simulink model "IEEE13NodeTestFeeder"  (R2023b)
settings: Solver=FixedStepAuto  StartTime=0.0  StopTime=3  FixedStep=0.004  MaxStep=0.04  RelTol=1e-3
PreLoadFcn:
  | IEEE13NodeTestFeederInit;
  | Ts=50e-6;
values from neighbouring files (symbols this model uses):
  C_601 = B_601/mi2km*ms2F    [IEEE13NodeTestFeederInit.m]
  C_602 = B_602/mi2km*ms2F    [IEEE13NodeTestFeederInit.m]
  C_603 = B_603/mi2km*ms2F    [IEEE13NodeTestFeederInit.m]
  C_604 = B_604/mi2km*ms2F    [IEEE13NodeTestFeederInit.m]
  C_605 = B_605/mi2km*ms2F    [IEEE13NodeTestFeederInit.m]
  C_606 = B_606/mi2km*ms2F    [IEEE13NodeTestFeederInit.m]
  C_607 = B_607/mi2km*ms2F    [IEEE13NodeTestFeederInit.m]
  ft2km = 0.0003048    [IEEE13NodeTestFeederInit.m]
  L_601 = X_601/mi2km/2/pi/60    [IEEE13NodeTestFeederInit.m]
  L_602 = X_602/mi2km/2/pi/60    [IEEE13NodeTestFeederInit.m]
  L_603 = X_603/mi2km/2/pi/60    [IEEE13NodeTestFeederInit.m]
  L_604 = X_604/mi2km/2/pi/60    [IEEE13NodeTestFeederInit.m]
  L_605 = X_605/mi2km/2/pi/60    [IEEE13NodeTestFeederInit.m]
  L_606 = X_606/mi2km/2/pi/60    [IEEE13NodeTestFeederInit.m]
  L_607 = X_607/mi2km/2/pi/60    [IEEE13NodeTestFeederInit.m]
  R_601 = R_601/mi2km    [IEEE13NodeTestFeederInit.m]
  R_602 = R_602/mi2km    [IEEE13NodeTestFeederInit.m]
  R_603 = R_603/mi2km    [IEEE13NodeTestFeederInit.m]
  R_604 = R_604/mi2km    [IEEE13NodeTestFeederInit.m]
  R_605 = R_605/mi2km    [IEEE13NodeTestFeederInit.m]
  R_606 = R_606/mi2km    [IEEE13NodeTestFeederInit.m]
  R_607 = R_607/mi2km    [IEEE13NodeTestFeederInit.m]
libraries: spsPowerPhasorLib x18, spsThreePhaseVIMeasurementLib x16, spsSeriesRLCLoadLib x12, spsLoadFlowBusLib x12, spsThreePhaseFaultLib x12, spsGroundLib x10, spsPiSectionLineLib x9, spsThreePhaseSeriesRLCLoadLib x8, spsMultimeterLib x6, spsThreePhaseSourceLib x1, spsThreePhaseBreakerLib x1, spsThreePhaseTransformerTwoWindingsLib x1
settings Model: Creator=The MathWorks, Inc.  LastModifiedBy=Dell
settings SolverCC: AlgebraicLoopSolver=TrustRegion
settings DataIOCC: ExternalInput=getinputstruct(op_IEEE_13_node_5)  InitialState=getstatestruct(op_IEEE_13_node_5)  LimitDataPoints=on  SaveFinalState=on  SaveOperatingPoint=on  SaveFormat=StructureWithTime  SaveState=on  LoggingToFile=on
settings OptimizationCC: LifeSpan=inf
settings DebuggingCC: AlgebraicLoopMsg=none  FcnCallInpInsideContextMsg=warning  StateNameClashWarn=warning  SFUnexpectedBacktrackingDiag=warning  SFNoUnconditionalDefaultTransitionDiag=warning  SFExecutionAtInitializationDiag=none
settings ModelReferenceCC: EnableRefExpFcnMdlSchedulingChecks=on  PropagateSignalLabelsOutOfModel=off
settings SFSimCC: CustomCodeUndefinedFunction=UseInterfaceOnly
settings CodeAppCC: StateflowObjectComments=on
settings SimscapeCC: SimscapeNormalizeSystem=off

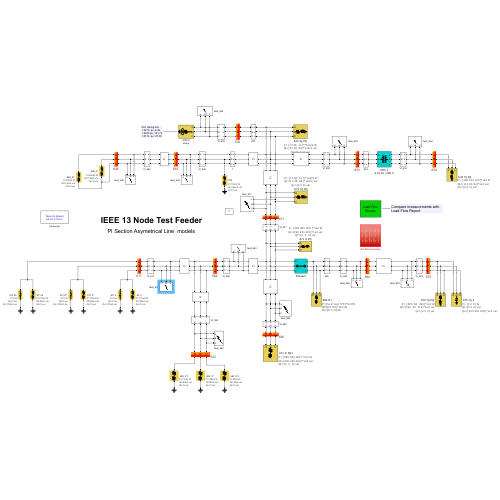
[thumbnail: Simulink's stored preview of the top-level diagram]
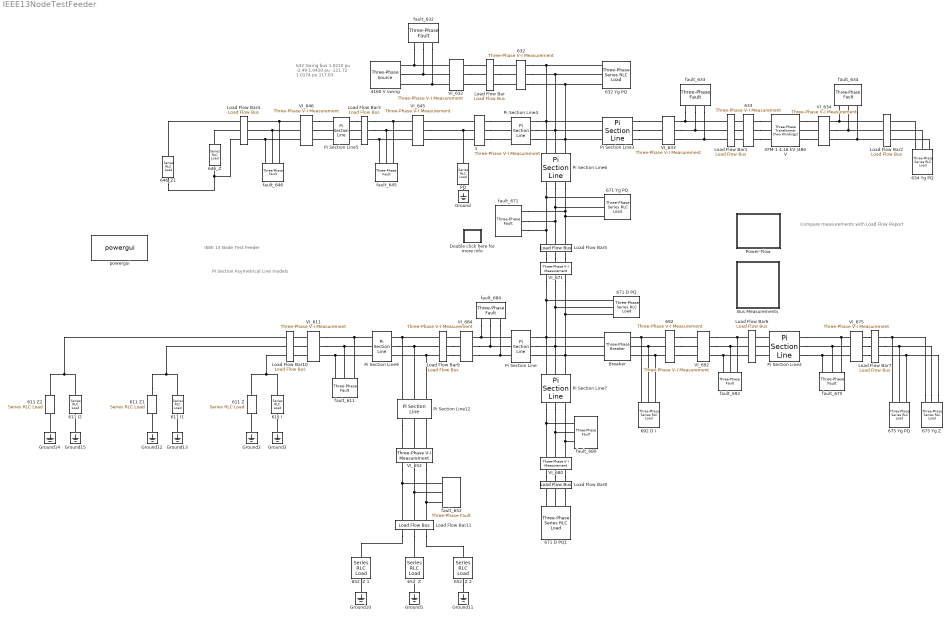
== system IEEE13NodeTestFeeder ==
  note: Compare measurements with
      | Load Flow Report
  note: 632 Swing bus
      | 1.0210 pu -2.49
      | 1.0420 pu -121.72
      | 1.0174 pu 117.83
  note: PI Section Asymetrical Line models
  note: IEEE 13 Node Test Feeder
  " 634 Yg PQ " : spsThreePhaseSeriesRLCLoadLib/Three-Phase Series RLC Load  LConnTagsString=A|B|C  Configuration=Y (grounded)  NominalVoltage=120e3  Vabc=[ 0.993926 1.02168 0.995885]*277.128  Vabcp=[1e3 1e3 1e3]  NominalFrequency=60  UnbalancedPower=on  ActivePower=1e+006  InductivePower=0  CapacitivePower=0  Pabc=[160 120 120]*1e3  QLabc=[110 90 90]*1e3  QCabc=[0 0 0]  Pabcp=[10e3 9e3 11e3]  QLabcp=[100 90 110]  QCabcp=[100 90 110]  Measurements=None  LoadType=constant PQ
      settings: AttributesFormatString=|
      | P= %<Pabc> W
      | Ql=%<QLabc> var
      | Qc=%<QCabc> var
  1 : spsThreePhaseVIMeasurementLib/Three-Phase V-I Measurement  VoltageMeasurement=phase-to-ground  SetLabelV=on  LabelV=Vabc_645  Vpu=off  VpuLL=off  CurrentMeasurement=yes  SetLabelI=on  LabelI=Iabc_645  Ipu=off  Pbase=100e6  Vbase=4160  OutputType=Complex  PhasorSimulation=on  PSBequivalent=0
  4160 V swing : spsThreePhaseSourceLib/Three-Phase Source  InternalConnection=Yg  VoltagePhases=on  Voltage=120e3  PhaseAngle=0  Voltage_phases=[ 1.021 1.042 1.0174]*2401.78  PhaseAngles_phases=[ -2.49006 -121.72 117.83]  Frequency=60  NonIdealSource=on  SpecifyImpedance=off  Resistance=1e-5  Inductance=0  ShortCircuitLevel=100e6  BaseVoltage=120e3  XRratio=10  BusType=swing  Pref=0  Qref=0  Prefabc=[0 0 0]  Qrefabc=[0 0 0]  Qmin="[-inf  -inf -inf]"  Qmax="[inf  inf inf]"
  611 I : spsSeriesRLCLoadLib/Series RLC Load  LConnTagsString=a  RConnTagsString=__new0  NominalVoltage=0.986755*2401.78  NominalFrequency=60  ActivePower=170e3  InductivePower=80e3  CapacitivePower=0  Setx0=off  InitialVoltage=0  SetiL0=off  InitialCurrent=0  Measurements=Branch voltage and current  LoadType=constant I
      settings: AttributesFormatString=|
      | P=%<ActivePower> W
      | Ql=%<InductivePower> var
      | Qc=%<CapacitivePower> var
  611 I1 : spsSeriesRLCLoadLib/Series RLC Load  LConnTagsString=a  RConnTagsString=__new0  NominalVoltage=0.986755*2401.78  NominalFrequency=60  ActivePower=170e3  InductivePower=80e3  CapacitivePower=0  Setx0=off  InitialVoltage=0  SetiL0=off  InitialCurrent=0  Measurements=Branch voltage and current  LoadType=constant PQ
      settings: AttributesFormatString=|
      | P=%<ActivePower> W
      | Ql=%<InductivePower> var
      | Qc=%<CapacitivePower> var
  611 I2 : spsSeriesRLCLoadLib/Series RLC Load  LConnTagsString=a  RConnTagsString=__new0  NominalVoltage=0.986755*2401.78  NominalFrequency=60  ActivePower=170e3  InductivePower=80e3  CapacitivePower=0  Setx0=off  InitialVoltage=0  SetiL0=off  InitialCurrent=0  Measurements=Branch voltage and current  LoadType=constant I
      settings: AttributesFormatString=|
      | P=%<ActivePower> W
      | Ql=%<InductivePower> var
      | Qc=%<CapacitivePower> var
  611 Z : spsSeriesRLCLoadLib/Series RLC Load  LConnTagsString=a  RConnTagsString=__new0  NominalVoltage=4160/sqrt(3)  NominalFrequency=60  ActivePower=0  InductivePower=0  CapacitivePower=100e3  Setx0=off  InitialVoltage=0  SetiL0=off  InitialCurrent=0  Measurements=None  LoadType=constant Z
      settings: AttributesFormatString=|
      | P=%<ActivePower> W
      | Ql=%<InductivePower> var
      | Qc=%<CapacitivePower> var
  611 Z1 : spsSeriesRLCLoadLib/Series RLC Load  LConnTagsString=a  RConnTagsString=__new0  NominalVoltage=4160/sqrt(3)  NominalFrequency=60  ActivePower=0  InductivePower=0  CapacitivePower=100e3  Setx0=off  InitialVoltage=0  SetiL0=off  InitialCurrent=0  Measurements=None  LoadType=constant I
      settings: AttributesFormatString=|
      | P=%<ActivePower> W
      | Ql=%<InductivePower> var
      | Qc=%<CapacitivePower> var
  611 Z2 : spsSeriesRLCLoadLib/Series RLC Load  LConnTagsString=a  RConnTagsString=__new0  NominalVoltage=4160/sqrt(3)  NominalFrequency=60  ActivePower=0  InductivePower=0  CapacitivePower=100e3  Setx0=off  InitialVoltage=0  SetiL0=off  InitialCurrent=0  Measurements=None  LoadType=constant PQ
      settings: AttributesFormatString=|
      | P=%<ActivePower> W
      | Ql=%<InductivePower> var
      | Qc=%<CapacitivePower> var
  632 : spsThreePhaseVIMeasurementLib/Three-Phase V-I Measurement  VoltageMeasurement=phase-to-ground  SetLabelV=on  LabelV=Vabc_632  Vpu=off  VpuLL=off  CurrentMeasurement=yes  SetLabelI=on  LabelI=Iabc_632  Ipu=off  Pbase=100e6  Vbase=4160  OutputType=Complex  PhasorSimulation=on  PSBequivalent=0
  632 Yg PQ : spsThreePhaseSeriesRLCLoadLib/Three-Phase Series RLC Load  LConnTagsString=A|B|C  Configuration=Y (grounded)  NominalVoltage=120e3  Vabc=[ 1.021 1.042 1.0174]*2401.78  Vabcp=[1e3 1e3 1e3]  NominalFrequency=60  UnbalancedPower=on  ActivePower=1e+006  InductivePower=0  CapacitivePower=0  Pabc="[17 66  117]*1e3/2"  QLabc="[10 38  68]*1e3/2"  QCabc=[0 0 0]  Pabcp=[10e3 9e3 11e3]  QLabcp=[100 90 110]  QCabcp=[100 90 110]  Measurements=None  LoadType=constant PQ
      settings: AttributesFormatString=|
      | P= %<Pabc> W
      | Ql=%<QLabc> var
      | Qc=%<QCabc> var
  633 : spsThreePhaseVIMeasurementLib/Three-Phase V-I Measurement  VoltageMeasurement=phase-to-ground  SetLabelV=on  LabelV=Vabc_633  Vpu=off  VpuLL=off  CurrentMeasurement=yes  SetLabelI=on  LabelI=Iabc_633  Ipu=off  Pbase=100e6  Vbase=4160  OutputType=Complex  PhasorSimulation=on  PSBequivalent=0
  646_Z : spsSeriesRLCLoadLib/Series RLC Load  LConnTagsString=a  RConnTagsString=__new0  NominalVoltage=4160  NominalFrequency=60  ActivePower=230e3  InductivePower=132e3  CapacitivePower=0  Setx0=off  InitialVoltage=0  SetiL0=off  InitialCurrent=0  Measurements=None  LoadType=constant Z
      settings: AttributesFormatString=|
      | P=%<ActivePower> W
      | Ql=%<InductivePower> var
      | Qc=%<CapacitivePower> var
  646_Z1 : spsSeriesRLCLoadLib/Series RLC Load  LConnTagsString=a  RConnTagsString=__new0  NominalVoltage=4160  NominalFrequency=60  ActivePower=230e3  InductivePower=132e3  CapacitivePower=0  Setx0=off  InitialVoltage=0  SetiL0=off  InitialCurrent=0  Measurements=None  LoadType=constant PQ
      settings: AttributesFormatString=|
      | P=%<ActivePower> W
      | Ql=%<InductivePower> var
      | Qc=%<CapacitivePower> var
  "652  Z " : spsSeriesRLCLoadLib/Series RLC Load  LConnTagsString=a  RConnTagsString=__new0  NominalVoltage=4160/sqrt(3)  NominalFrequency=60  ActivePower=128e3  InductivePower=86e3  CapacitivePower=0  Setx0=off  InitialVoltage=0  SetiL0=off  InitialCurrent=0  Measurements=None  LoadType=constant Z
      settings: AttributesFormatString=|
      | P=%<ActivePower> W
      | Ql=%<InductivePower> var
      | Qc=%<CapacitivePower> var
  652  Z 1 : spsSeriesRLCLoadLib/Series RLC Load  LConnTagsString=a  RConnTagsString=__new0  NominalVoltage=4160/sqrt(3)  NominalFrequency=60  ActivePower=115e3  InductivePower=80e3  CapacitivePower=0  Setx0=off  InitialVoltage=0  SetiL0=off  InitialCurrent=0  Measurements=None  LoadType=constant PQ
      settings: AttributesFormatString=|
      | P=%<ActivePower> W
      | Ql=%<InductivePower> var
      | Qc=%<CapacitivePower> var
  652  Z 2 : spsSeriesRLCLoadLib/Series RLC Load  LConnTagsString=a  RConnTagsString=__new0  NominalVoltage=4160/sqrt(3)  NominalFrequency=60  ActivePower=80e3  InductivePower=43e3  CapacitivePower=0  Setx0=off  InitialVoltage=0  SetiL0=off  InitialCurrent=0  Measurements=None  LoadType=constant I
      settings: AttributesFormatString=|
      | P=%<ActivePower> W
      | Ql=%<InductivePower> var
      | Qc=%<CapacitivePower> var
  671 D PQ : spsThreePhaseSeriesRLCLoadLib/Three-Phase Series RLC Load  LConnTagsString=A|B|C  Configuration=Delta  NominalVoltage=120e3  Vabc="[1  1  1]*120e3/sqrt(3)"  Vabcp=[ 1.7426 1.77325 1.71534]*2401.78  NominalFrequency=60  UnbalancedPower=on  ActivePower=1e+006  InductivePower=0  CapacitivePower=0  Pabc="[17 66  117]*1e3/2"  QLabc="[10 38  68]*1e3/2"  QCabc=[0 0 0]  Pabcp=[385 385 385 ]*1e3  QLabcp=[220 220 220]*1e3  QCabcp="[0  0  0]"  Measurements=Branch voltages and currents  LoadType=constant PQ
      settings: AttributesFormatString=|
      | P= %<Pabcp> W
      | Ql=%<QLabcp> var
      | Qc=%<QCabcp> var
  671 D PQ1 : spsThreePhaseSeriesRLCLoadLib/Three-Phase Series RLC Load  LConnTagsString=A|B|C  Configuration=Delta  NominalVoltage=120e3  Vabc="[1  1  1]*120e3/sqrt(3)"  Vabcp=[ 1.7426 1.77325 1.71534]*2401.78  NominalFrequency=60  UnbalancedPower=on  ActivePower=1e+006  InductivePower=0  CapacitivePower=0  Pabc="[17 66  117]*1e3/2"  QLabc="[10 38  68]*1e3/2"  QCabc=[0 0 0]  Pabcp=[385 385 385 ]*1e3  QLabcp=[220 220 220]*1e3  QCabcp="[0  0  0]"  Measurements=Branch voltages and currents  LoadType=constant Z
      settings: AttributesFormatString=|
      | P= %<Pabcp> W
      | Ql=%<QLabcp> var
      | Qc=%<QCabcp> var
  671 Yg PQ : spsThreePhaseSeriesRLCLoadLib/Three-Phase Series RLC Load  LConnTagsString=A|B|C  Configuration=Y (grounded)  NominalVoltage=120e3  Vabc=[ 0.990007 1.05293 0.977696]*2401.78  Vabcp=[1e3 1e3 1e3]  NominalFrequency=60  UnbalancedPower=on  ActivePower=1e+006  InductivePower=0  CapacitivePower=0  Pabc="[17 66  117]*1e3/2"  QLabc="[10 38  68]*1e3/2"  QCabc=[0 0 0]  Pabcp=[10e3 9e3 11e3]  QLabcp=[100 90 110]  QCabcp=[100 90 110]  Measurements=None  LoadType=constant PQ
      settings: AttributesFormatString=|
      | P= %<Pabc> W
      | Ql=%<QLabc> var
      | Qc=%<QCabc> var
  675 Yg PQ : spsThreePhaseSeriesRLCLoadLib/Three-Phase Series RLC Load  LConnTagsString=A|B|C  Configuration=Y (grounded)  NominalVoltage=120e3  Vabc=[ 0.983621 1.05532 0.975578]*2401.78  Vabcp=[1e3 1e3 1e3]  NominalFrequency=60  UnbalancedPower=on  ActivePower=1e+006  InductivePower=0  CapacitivePower=0  Pabc="[485  68  290]*1e3"  QLabc="[190  60  212]*1e3"  QCabc=[0 0 0]  Pabcp=[10e3 9e3 11e3]  QLabcp=[100 90 110]  QCabcp=[100 90 110]  Measurements=Branch voltages and currents  LoadType=constant PQ
      settings: AttributesFormatString=|
      | P= %<Pabc> W
      | Ql=%<QLabc> var
      | Qc=%<QCabc> var
  675 Yg Z : spsThreePhaseSeriesRLCLoadLib/Three-Phase Series RLC Load  LConnTagsString=A|B|C  Configuration=Y (grounded)  NominalVoltage=120e3  Vabc="[1  1  1]*4160/sqrt(3)"  Vabcp=[1e3 1e3 1e3]  NominalFrequency=60  UnbalancedPower=on  ActivePower=1e+006  InductivePower=0  CapacitivePower=0  Pabc=[0 0 0]  QLabc=[0 0 0]  QCabc=[200 200 200]*1e3  Pabcp=[10e3 9e3 11e3]  QLabcp=[100 90 110]  QCabcp=[100 90 110]  Measurements=None  LoadType=constant Z
      settings: AttributesFormatString=|
      | P= %<Pabc> W
      | Ql=%<QLabc> var
      | Qc=%<QCabc> var
  692 : spsThreePhaseVIMeasurementLib/Three-Phase V-I Measurement  VoltageMeasurement=phase-to-ground  SetLabelV=on  LabelV=Vabc_692  Vpu=off  VpuLL=off  CurrentMeasurement=yes  SetLabelI=on  LabelI=Iabc_692  Ipu=off  Pbase=100e6  Vbase=4160  OutputType=Complex  PhasorSimulation=on  PSBequivalent=0
  692 D I : spsThreePhaseSeriesRLCLoadLib/Three-Phase Series RLC Load  LConnTagsString=A|B|C  Configuration=Delta  NominalVoltage=120e3  Vabc="[1  1  1]*120e3/sqrt(3)"  Vabcp=[ 1.73731 1.75253 1.72367]*2401.78  NominalFrequency=60  UnbalancedPower=on  ActivePower=1e+006  InductivePower=0  CapacitivePower=0  Pabc="[17 66  117]*1e3/2"  QLabc="[10 38  68]*1e3/2"  QCabc=[0 0 0]  Pabcp=[1e-6 1e-6 170 ]*1e3  QLabcp=[0 0 151]*1e3  QCabcp="[0  0  0]"  Measurements=Branch voltages and currents  LoadType=constant I
      settings: AttributesFormatString=|
      | P= %<Pabcp> W
      | Ql=%<QLabcp> var
      | Qc=%<QCabcp> var
  Breaker : spsThreePhaseBreakerLib/Three-Phase Breaker  InitialState=closed  SwitchA=off  SwitchB=off  SwitchC=off  SwitchTimes=[0.5 ]  External=off  BreakerResistance=0.0001  SnubberResistance=inf  SnubberCapacitance=0  Measurements=None
  Bus Measurements : Subsystem
  Double click here for more info : Subsystem
      settings: OpenFcn="showExample(\"simscapeelectricalsps/IEEE13NodeTestFeederExample\")"
      mask Display: disp('?')
  Ground{,1..3,10..15} (10 alike) : spsGroundLib/Ground  LConnTagsString=a
  Load Flow Bar : spsLoadFlowBusLib/Load Flow Bus  LConnTagsString=a|b|c  RConnTagsString=a|b|c  Phases=ABC  Connectors=on both sides  ID=632  Vbase=4160/sqrt(3)  Vref="[ 1.0210  1.0420  1.0174]"  Vangle="[ -2.49  -121.72  117.83]"  VLF=1.021  VLFb=1.042  VLFc=1.017  angleLF=-2.49  angleLFb=-121.7  angleLFc=117.8
      settings: AttributesFormatString=%<ID>
  Load Flow Bar1 : spsLoadFlowBusLib/Load Flow Bus  LConnTagsString=a|b|c  RConnTagsString=a|b|c  Phases=ABC  Connectors=on both sides  ID=633  Vbase=4160/sqrt(3)  Vref=[1.0 1.0 1.0]  Vangle=[0 -120 120]  VLF=1.018  VLFb=1.04  VLFc=1.015  angleLF=-2.555  angleLFb=-121.8  angleLFc=117.8
      settings: AttributesFormatString=%<ID>
  Load Flow Bar10 : spsLoadFlowBusLib/Load Flow Bus  LConnTagsString=a|b|c  RConnTagsString=a|b|c  Phases=ABC  Connectors=on both sides  ID=611  Vbase=4160/sqrt(3)  Vref=[1.0 1.0 1.0]  Vangle=[0 -120, 120]  VLF=NaN  VLFb=NaN  VLFc=0.9737  angleLF=NaN  angleLFb=NaN  angleLFc=115.8
      settings: AttributesFormatString=%<ID>
  Load Flow Bar11 : spsLoadFlowBusLib/Load Flow Bus  LConnTagsString=a|b|c  RConnTagsString=a|b|c  Phases=ABC  Connectors=on both sides  ID=652  Vbase=4160/sqrt(3)  Vref=[1.0 1.0 1.0]  Vangle=[0 -120 120]  VLF=0.9825  VLFb=NaN  VLFc=NaN  angleLF=-5.246  angleLFb=NaN  angleLFc=NaN
      settings: AttributesFormatString=%<ID>
  Load Flow Bar2 : spsLoadFlowBusLib/Load Flow Bus  LConnTagsString=a|b|c  RConnTagsString=a|b|c  Phases=ABC  Connectors=on both sides  ID=634  Vbase=480/sqrt(3)  Vref=[1.0 1.0 1.0]  Vangle=[0 -120 120]  VLF=0.9939  VLFb=1.022  VLFc=0.9959  angleLF=-3.232  angleLFb=-122.2  angleLFc=117.3
      settings: AttributesFormatString=%<ID>
  Load Flow Bar3 : spsLoadFlowBusLib/Load Flow Bus  LConnTagsString=a|b|c  RConnTagsString=a|b|c  Phases=ABC  Connectors=on both sides  ID=645  Vbase=4160/sqrt(3)  Vref=[1.0 1.0 1.0]  Vangle=[0 0 0]  VLF=NaN  VLFb=1.033  VLFc=1.015  angleLF=NaN  angleLFb=-121.9  angleLFc=117.9
      settings: AttributesFormatString=%<ID>
  Load Flow Bar4 : spsLoadFlowBusLib/Load Flow Bus  LConnTagsString=a|b|c  RConnTagsString=a|b|c  Phases=ABC  Connectors=on both sides  ID=646  Vbase=4160/sqrt(3)  Vref=[1.0 1.0 1.0]  Vangle=[0 0 0]  VLF=NaN  VLFb=1.031  VLFc=1.013  angleLF=NaN  angleLFb=-122  angleLFc=117.9
      settings: AttributesFormatString=%<ID>
  Load Flow Bar5 : spsLoadFlowBusLib/Load Flow Bus  LConnTagsString=a|b|c  RConnTagsString=a|b|c  Phases=ABC  Connectors=on both sides  ID=671  Vbase=4160/sqrt(3)  Vref=[1.0 1.0 1.0]  Vangle=[0 -120 120]  VLF=0.99  VLFb=1.053  VLFc=0.9777  angleLF=-5.298  angleLFb=-122.3  angleLFc=116
      settings: AttributesFormatString=%<ID>
  Load Flow Bar6 : spsLoadFlowBusLib/Load Flow Bus  LConnTagsString=a|b|c  RConnTagsString=a|b|c  Phases=ABC  Connectors=on both sides  ID=692  Vbase=4160/sqrt(3)  Vref=[1.0 1.0 1.0]  Vangle=[0 -120 120]  VLF=0.99  VLFb=1.053  VLFc=0.9777  angleLF=-5.298  angleLFb=-122.3  angleLFc=116
      settings: AttributesFormatString=%<ID>
  Load Flow Bar7 : spsLoadFlowBusLib/Load Flow Bus  LConnTagsString=a|b|c  RConnTagsString=a|b|c  Phases=ABC  Connectors=on both sides  ID=675  Vbase=4160/sqrt(3)  Vref=[1.0 1.0 1.0]  Vangle=[0 -120 120]  VLF=0.9836  VLFb=1.055  VLFc=0.9756  angleLF=-5.544  angleLFb=-122.5  angleLFc=116
      settings: AttributesFormatString=%<ID>
  Load Flow Bar8 : spsLoadFlowBusLib/Load Flow Bus  LConnTagsString=a|b|c  RConnTagsString=a|b|c  Phases=ABC  Connectors=on both sides  ID=680  Vbase=4160/sqrt(3)  Vref=[1.0 1.0 1.0]  Vangle=[0 -120 120]  VLF=0.99  VLFb=1.053  VLFc=0.9777  angleLF=-5.298  angleLFb=-122.3  angleLFc=116
      settings: AttributesFormatString=%<ID>
  Load Flow Bar9 : spsLoadFlowBusLib/Load Flow Bus  LConnTagsString=a|b|c  RConnTagsString=a|b|c  Phases=ABC  Connectors=on both sides  ID=684  Vbase=4160/sqrt(3)  Vref=[1.0 1.0 1.0]  Vangle=[0 -120 120]  VLF=0.9881  VLFb=NaN  VLFc=0.9757  angleLF=-5.321  angleLFb=NaN  angleLFc=115.9
      settings: AttributesFormatString=%<ID>
  PQ : spsSeriesRLCLoadLib/Series RLC Load  LConnTagsString=a  RConnTagsString=__new0  NominalVoltage=1.03283*2401.78  NominalFrequency=60  ActivePower=170e3  InductivePower=125e3  CapacitivePower=0  Setx0=off  InitialVoltage=0  SetiL0=off  InitialCurrent=0  Measurements=None  LoadType=constant PQ
      settings: AttributesFormatString=|
      | P=%<ActivePower> W
      | Ql=%<InductivePower> var
      | Qc=%<CapacitivePower> var
  Pi Section Line : spsPiSectionLineLib/Pi Section Line  LConnTagsString=1|i2|i3  RConnTagsString=1|o2|o3  Phases=3  PiSections=1  Length=300*ft2km  Frequency=60  Resistance=R_604  Inductance=L_604  Capacitance=C_604  SpecifyConductance=off  Conductance=0  Measurements=None  Measurements2=None
      settings: LibrarySourceBlock=sps_lib/Power Grid Elements/Pi Section Line
  Pi Section Line12 : spsPiSectionLineLib/Pi Section Line  LConnTagsString=1|i2|i3  RConnTagsString=1|o2|o3  Phases=3  PiSections=1  Length=800*ft2km  Frequency=60  Resistance=R_607  Inductance=L_607  Capacitance=C_607  SpecifyConductance=off  Conductance=0  Measurements=None  Measurements2=None
      settings: LibrarySourceBlock=sps_lib/Power Grid Elements/Pi Section Line
  Pi Section Line2 : spsPiSectionLineLib/Pi Section Line  LConnTagsString=1|i2|i3  RConnTagsString=1|o2|o3  Phases=3  PiSections=1  Length=500*ft2km  Frequency=60  Resistance=R_606  Inductance=L_606  Capacitance=C_606  SpecifyConductance=off  Conductance=0  Measurements=None  Measurements2=None
      settings: LibrarySourceBlock=sps_lib/Power Grid Elements/Pi Section Line
  Pi Section Line3 : spsPiSectionLineLib/Pi Section Line  LConnTagsString=1|i2|i3  RConnTagsString=1|o2|o3  Phases=3  PiSections=1  Length=500*ft2km  Frequency=60  Resistance=R_602  Inductance=L_602  Capacitance=C_602  SpecifyConductance=off  Conductance=0  Measurements=None  Measurements2=None
      settings: LibrarySourceBlock=sps_lib/Power Grid Elements/Pi Section Line
  Pi Section Line4 : spsPiSectionLineLib/Pi Section Line  LConnTagsString=1|i2|i3  RConnTagsString=1|o2|o3  Phases=3  PiSections=1  Length=500*ft2km  Frequency=60  Resistance=R_603  Inductance=L_603  Capacitance=C_603  SpecifyConductance=off  Conductance=0  Measurements=None  Measurements2=None
      settings: LibrarySourceBlock=sps_lib/Power Grid Elements/Pi Section Line
  Pi Section Line5 : spsPiSectionLineLib/Pi Section Line  LConnTagsString=1|i2|i3  RConnTagsString=1|o2|o3  Phases=3  PiSections=1  Length=300*ft2km  Frequency=60  Resistance=R_603  Inductance=L_603  Capacitance=C_603  SpecifyConductance=off  Conductance=0  Measurements=None  Measurements2=None
      settings: LibrarySourceBlock=sps_lib/Power Grid Elements/Pi Section Line
  Pi Section Line6 : spsPiSectionLineLib/Pi Section Line  LConnTagsString=1|i2|i3  RConnTagsString=1|o2|o3  Phases=3  PiSections=1  Length=2000*ft2km  Frequency=60  Resistance=R_601  Inductance=L_601  Capacitance=C_601  SpecifyConductance=off  Conductance=0  Measurements=None  Measurements2=None
      settings: LibrarySourceBlock=sps_lib/Power Grid Elements/Pi Section Line
  Pi Section Line7 : spsPiSectionLineLib/Pi Section Line  LConnTagsString=1|i2|i3  RConnTagsString=1|o2|o3  Phases=3  PiSections=1  Length=1000*ft2km  Frequency=60  Resistance=R_601  Inductance=L_601  Capacitance=C_601  SpecifyConductance=off  Conductance=0  Measurements=None  Measurements2=None
      settings: LibrarySourceBlock=sps_lib/Power Grid Elements/Pi Section Line
  Pi Section Line9 : spsPiSectionLineLib/Pi Section Line  LConnTagsString=1|i2|i3  RConnTagsString=1|o2|o3  Phases=3  PiSections=1  Length=300*ft2km  Frequency=60  Resistance=R_605  Inductance=L_605  Capacitance=C_605  SpecifyConductance=off  Conductance=0  Measurements=None  Measurements2=None
      settings: LibrarySourceBlock=sps_lib/Power Grid Elements/Pi Section Line
  Power-Flow : Subsystem
      mask Display: disp('Load Flow\nResults')
  VI_611 : spsThreePhaseVIMeasurementLib/Three-Phase V-I Measurement  VoltageMeasurement=phase-to-ground  SetLabelV=on  LabelV=Bus611_Voltages  Vpu=off  VpuLL=off  CurrentMeasurement=yes  SetLabelI=on  LabelI=Bus611_Currents  Ipu=off  Pbase=100e6  Vbase=500e3  OutputType=Complex  PhasorSimulation=on  PSBequivalent=0
  VI_632 : spsThreePhaseVIMeasurementLib/Three-Phase V-I Measurement  VoltageMeasurement=phase-to-ground  SetLabelV=on  LabelV=Bus632_Voltages  Vpu=off  VpuLL=off  CurrentMeasurement=yes  SetLabelI=on  LabelI=Bus632_Currents  Ipu=off  Pbase=100e6  Vbase=500e3  OutputType=Complex  PhasorSimulation=on  PSBequivalent=0
  VI_633 : spsThreePhaseVIMeasurementLib/Three-Phase V-I Measurement  VoltageMeasurement=phase-to-ground  SetLabelV=on  LabelV=Bus633_Voltages  Vpu=off  VpuLL=off  CurrentMeasurement=yes  SetLabelI=on  LabelI=Bus633_Currents  Ipu=off  Pbase=100e6  Vbase=500e3  OutputType=Complex  PhasorSimulation=on  PSBequivalent=0
  VI_634 : spsThreePhaseVIMeasurementLib/Three-Phase V-I Measurement  VoltageMeasurement=phase-to-ground  SetLabelV=on  LabelV=Bus634_Voltages  Vpu=off  VpuLL=off  CurrentMeasurement=yes  SetLabelI=on  LabelI=Bus634_Currents  Ipu=off  Pbase=100e6  Vbase=500e3  OutputType=Complex  PhasorSimulation=on  PSBequivalent=0
  VI_645 : spsThreePhaseVIMeasurementLib/Three-Phase V-I Measurement  VoltageMeasurement=phase-to-ground  SetLabelV=on  LabelV=Bus645_Voltages  Vpu=off  VpuLL=off  CurrentMeasurement=yes  SetLabelI=on  LabelI=Bus645_Currents  Ipu=off  Pbase=100e6  Vbase=500e3  OutputType=Complex  PhasorSimulation=on  PSBequivalent=0
  VI_646 : spsThreePhaseVIMeasurementLib/Three-Phase V-I Measurement  VoltageMeasurement=phase-to-ground  SetLabelV=on  LabelV=Bus646_Voltages  Vpu=off  VpuLL=off  CurrentMeasurement=yes  SetLabelI=on  LabelI=Bus646_Currents  Ipu=off  Pbase=100e6  Vbase=500e3  OutputType=Complex  PhasorSimulation=on  PSBequivalent=0
  VI_652 : spsThreePhaseVIMeasurementLib/Three-Phase V-I Measurement  VoltageMeasurement=phase-to-ground  SetLabelV=on  LabelV=Bus652_Voltages  Vpu=off  VpuLL=off  CurrentMeasurement=yes  SetLabelI=on  LabelI=Bus652_Currents  Ipu=off  Pbase=100e6  Vbase=500e3  OutputType=Complex  PhasorSimulation=on  PSBequivalent=0
  VI_671 : spsThreePhaseVIMeasurementLib/Three-Phase V-I Measurement  VoltageMeasurement=phase-to-ground  SetLabelV=on  LabelV=Bus671_Voltages  Vpu=off  VpuLL=off  CurrentMeasurement=yes  SetLabelI=on  LabelI=Bus671_Currents  Ipu=off  Pbase=100e6  Vbase=500e3  OutputType=Complex  PhasorSimulation=on  PSBequivalent=0
  VI_675 : spsThreePhaseVIMeasurementLib/Three-Phase V-I Measurement  VoltageMeasurement=phase-to-ground  SetLabelV=on  LabelV=Bus675_Voltages  Vpu=off  VpuLL=off  CurrentMeasurement=yes  SetLabelI=on  LabelI=Bus675_Currents  Ipu=off  Pbase=100e6  Vbase=500e3  OutputType=Complex  PhasorSimulation=on  PSBequivalent=0
  VI_680 : spsThreePhaseVIMeasurementLib/Three-Phase V-I Measurement  VoltageMeasurement=phase-to-ground  SetLabelV=on  LabelV=Bus680_Voltages  Vpu=off  VpuLL=off  CurrentMeasurement=yes  SetLabelI=on  LabelI=Bus680_Currents  Ipu=off  Pbase=100e6  Vbase=500e3  OutputType=Complex  PhasorSimulation=on  PSBequivalent=0
  VI_684 : spsThreePhaseVIMeasurementLib/Three-Phase V-I Measurement  VoltageMeasurement=phase-to-ground  SetLabelV=on  LabelV=Bus684_Voltages  Vpu=off  VpuLL=off  CurrentMeasurement=yes  SetLabelI=on  LabelI=Bus684_Currents  Ipu=off  Pbase=100e6  Vbase=500e3  OutputType=Complex  PhasorSimulation=on  PSBequivalent=0
  VI_692 : spsThreePhaseVIMeasurementLib/Three-Phase V-I Measurement  VoltageMeasurement=phase-to-ground  SetLabelV=on  LabelV=Bus692_Voltages  Vpu=off  VpuLL=off  CurrentMeasurement=yes  SetLabelI=on  LabelI=Bus692_Currents  Ipu=off  Pbase=100e6  Vbase=500e3  OutputType=Complex  PhasorSimulation=on  PSBequivalent=0
  XFM-1 4.16 kV /480 V : spsThreePhaseTransformerTwoWindingsLib/Three-Phase Transformer (Two Windings)  Winding1Connection=Yg  Winding2Connection=Yg  CoreType=Three single-phase transformers  SetSaturation=off  Hysteresis=off  DataFile='hysteresis'  SetInitialFlux=off  Measurements=None  UNITS=pu  NominalPower=[ 500e3 , 60 ]  Winding1=[4160 0.011 0.02]  Winding2=[480 0 0]  Rm=500  Lm=500  L0=0.5  Saturation=[0 0;0.0024 1.2;1 1.52]  InitialFluxes=[0.8 -0.8 0.7]  BreakLoop=off  DiscreteSolver=Trapezoidal iterative  DataType=off  TransfoNumber=1
  fault_{611,645..646,652,671,675,680,684} (8 alike) : spsThreePhaseFaultLib/Three-Phase Fault  InitialStates=0  FaultA=off  FaultB=off  FaultC=off  GroundFault=off  SwitchTimes=[0 4]  External=off  SwitchStatus=NaN  FaultResistance=0.01  GroundResistance=0.01  SnubberResistance=1e6  SnubberCapacitance=inf  Measurements=None
  fault_{632..634,692} (4 alike) : spsThreePhaseFaultLib/Three-Phase Fault  InitialStates=0  FaultA=off  FaultB=off  FaultC=off  GroundFault=off  SwitchTimes=[0.5 2]  External=off  SwitchStatus=NaN  FaultResistance=0.01  GroundResistance=0.01  SnubberResistance=1e6  SnubberCapacitance=inf  Measurements=None
  powergui : spspowerguiLib/powergui  Priority=1  SimulationMode=Discrete phasor  SampleTime=4e-3  frequency=60  Iterations=50  frequencyindice=60  Pbase=100e3  ErrMax=0.0001  UnitsV=kV  UnitsW=kW  buscounter=0  FunctionMessages=off  echomessages=off  EnableUseOfTLC=off  CurrentSourceSwitches=off  DisableSnubberDevices=off  DisableRonSwitches=off  DisableVfSwitches=off  DisplayEquations=off  AutomaticDiscreteSolvers=off  SolverType=Tustin/Backward Euler (TBE)  Interpol=off  ExternalGateDelay=off  methode=off  Ts=0  x0status=blocks  SPID=off  SwTol=0  HookPort=off  NonlinearTolerance=1e-4  nMaxIteration=100  ContinueOnMaxIteration=off  RestoreLinks=warning  ResistiveCurrentMeasurement=off  Frange=[0:2:500]  Ylog=off  Xlog=on  ShowGrid=off  save=off  variable=ZData  structure=0  ZoomFFT=on  StartTime=0.0  cycles=1  DisplayStyle=1  fundamental=60  FreqAxis=off  MaxFrequency=1000  frequencyindicesteady=1  RmsSteady=1  display=off
  connections:
  632/RConn2 -- 632 Yg PQ/LConn2 -- Pi Section Line4/RConn2 -- Pi Section Line6/LConn2 -- Pi Section Line3/LConn2
  675 Yg Z/LConn1 -- Load Flow Bar7/LConn1 -- 675 Yg PQ/LConn1
  671 D PQ/LConn2 -- VI_671/LConn2 -- Pi Section Line/RConn2 -- Breaker/LConn2 -- Pi Section Line7/LConn2
  Breaker/RConn3 -- 692 D I/LConn3 -- 692/LConn3
  Pi Section Line7/LConn1 -- Pi Section Line/RConn1 -- VI_671/LConn1 -- 671 D PQ/LConn1 -- Breaker/LConn1
  PQ/LConn1 -- 1/LConn2 -- VI_645/RConn2
  675 Yg Z/LConn3 -- Load Flow Bar7/LConn3 -- 675 Yg PQ/LConn3
  671 Yg PQ/LConn2 -- Load Flow Bar5/LConn2 -- fault_671/LConn2 -- Pi Section Line6/RConn2
  611 I/LConn1 -- Load Flow Bar10/LConn3 -- 611 Z/LConn1
  671 Yg PQ/LConn3 -- Pi Section Line6/RConn3 -- fault_671/LConn3 -- Load Flow Bar5/LConn3
  Pi Section Line6/LConn1 -- Pi Section Line4/RConn1 -- 632 Yg PQ/LConn1 -- 632/RConn1 -- Pi Section Line3/LConn1
  671 D PQ/LConn3 -- VI_671/LConn3 -- Pi Section Line/RConn3 -- Pi Section Line7/LConn3 -- Breaker/LConn3
  632/RConn3 -- 632 Yg PQ/LConn3 -- Pi Section Line4/RConn3 -- Pi Section Line6/LConn3 -- Pi Section Line3/LConn3
  Breaker/RConn1 -- 692 D I/LConn1 -- 692/LConn1
  671 Yg PQ/LConn1 -- Load Flow Bar5/LConn1 -- fault_671/LConn1 -- Pi Section Line6/RConn1
  Breaker/RConn2 -- 692 D I/LConn2 -- 692/LConn2
  675 Yg Z/LConn2 -- Load Flow Bar7/LConn2 -- 675 Yg PQ/LConn2
  fault_692/LConn1 -- VI_692/RConn1 -- Load Flow Bar6/RConn1
  Ground2/LConn1 -- 611 Z/RConn1
  fault_692/LConn3 -- VI_692/RConn3 -- Load Flow Bar6/RConn3
  " 634 Yg PQ "/LConn2 -- Load Flow Bar2/RConn2
  Pi Section Line2/RConn3 -- fault_675/LConn3 -- VI_675/LConn3
  Pi Section Line7/RConn3 -- fault_680/LConn3 -- VI_680/RConn3
  633/LConn1 -- Load Flow Bar1/RConn1
  Pi Section Line2/RConn1 -- fault_675/LConn1 -- VI_675/LConn1
  Ground/LConn1 -- PQ/RConn1
  Pi Section Line7/RConn1 -- fault_680/LConn1 -- VI_680/RConn1
  Load Flow Bar4/LConn3 -- 646_Z1/RConn1 -- 646_Z/RConn1
  1/RConn3 -- Pi Section Line4/LConn3
  Pi Section Line7/RConn2 -- fault_680/LConn2 -- VI_680/RConn2
  fault_692/LConn2 -- VI_692/RConn2 -- Load Flow Bar6/RConn2
  Ground1/LConn1 -- "652  Z "/RConn1
  Pi Section Line2/LConn1 -- Load Flow Bar6/LConn1
  633/RConn3 -- XFM-1 4.16 kV /480 V/LConn3
  633/RConn2 -- XFM-1 4.16 kV /480 V/LConn2
  1/RConn1 -- Pi Section Line4/LConn1
  633/RConn1 -- XFM-1 4.16 kV /480 V/LConn1
  Pi Section Line2/LConn2 -- Load Flow Bar6/LConn2
  Load Flow Bar/RConn2 -- 632/LConn2
  Ground3/LConn1 -- 611 I/RConn1
  Load Flow Bar/RConn1 -- 632/LConn1
  Pi Section Line2/RConn2 -- fault_675/LConn2 -- VI_675/LConn2
  633/LConn3 -- Load Flow Bar1/RConn3
  Load Flow Bar/RConn3 -- 632/LConn3
  633/LConn2 -- Load Flow Bar1/RConn2
  1/LConn1 -- VI_645/RConn1
  Pi Section Line9/RConn2 -- Load Flow Bar9/LConn2 -- Pi Section Line12/LConn2
  " 634 Yg PQ "/LConn1 -- Load Flow Bar2/RConn1
  Pi Section Line2/LConn3 -- Load Flow Bar6/LConn3
  1/RConn2 -- Pi Section Line4/LConn2
  " 634 Yg PQ "/LConn3 -- Load Flow Bar2/RConn3
  646_Z/LConn1 -- Load Flow Bar4/LConn2
  VI_632/RConn1 -- Load Flow Bar/LConn1
  VI_632/RConn2 -- Load Flow Bar/LConn2
  VI_632/RConn3 -- Load Flow Bar/LConn3
  VI_632/LConn1 -- fault_632/LConn1 -- 4160 V swing/RConn1
  VI_632/LConn2 -- fault_632/LConn2 -- 4160 V swing/RConn2
  VI_632/LConn3 -- fault_632/LConn3 -- 4160 V swing/RConn3
  Pi Section Line3/RConn1 -- VI_633/LConn1
  Pi Section Line3/RConn2 -- VI_633/LConn2
  Pi Section Line3/RConn3 -- VI_633/LConn3
  VI_633/RConn1 -- Load Flow Bar1/LConn1 -- fault_633/LConn1
  VI_633/RConn2 -- Load Flow Bar1/LConn2 -- fault_633/LConn2
  VI_633/RConn3 -- Load Flow Bar1/LConn3 -- fault_633/LConn3
  XFM-1 4.16 kV /480 V/RConn1 -- VI_634/LConn1
  VI_634/LConn2 -- XFM-1 4.16 kV /480 V/RConn2
  XFM-1 4.16 kV /480 V/RConn3 -- VI_634/LConn3
  VI_634/RConn1 -- Load Flow Bar2/LConn1 -- fault_634/LConn1
  VI_634/RConn2 -- Load Flow Bar2/LConn2 -- fault_634/LConn2
  VI_634/RConn3 -- Load Flow Bar2/LConn3 -- fault_634/LConn3
  Pi Section Line5/LConn2 -- VI_646/RConn2
  Pi Section Line5/LConn3 -- VI_646/RConn3
  VI_646/LConn2 -- Load Flow Bar4/RConn2 -- fault_646/LConn2
  fault_646/LConn3 -- VI_646/LConn3 -- Load Flow Bar4/RConn3
  Load Flow Bar3/LConn2 -- Pi Section Line5/RConn2
  Pi Section Line5/RConn3 -- Load Flow Bar3/LConn3
  VI_645/RConn3 -- 1/LConn3
  VI_645/LConn2 -- Load Flow Bar3/RConn2 -- fault_645/LConn2
  VI_645/LConn3 -- Load Flow Bar3/RConn3 -- fault_645/LConn3
  fault_645/LConn1 -- Load Flow Bar3/RConn1 -- VI_645/LConn1
  fault_646/LConn1 -- VI_646/LConn1 -- Load Flow Bar4/RConn1
  Load Flow Bar5/RConn1 -- VI_671/RConn1
  Load Flow Bar5/RConn2 -- VI_671/RConn2
  Load Flow Bar5/RConn3 -- VI_671/RConn3
  VI_684/LConn1 -- Load Flow Bar9/RConn1
  VI_680/LConn1 -- Load Flow Bar8/LConn1
  VI_680/LConn2 -- Load Flow Bar8/LConn2
  VI_680/LConn3 -- Load Flow Bar8/LConn3
  692/RConn1 -- VI_692/LConn1
  692/RConn2 -- VI_692/LConn2
  692/RConn3 -- VI_692/LConn3
  VI_675/RConn1 -- Load Flow Bar7/RConn1
  VI_675/RConn2 -- Load Flow Bar7/RConn2
  VI_675/RConn3 -- Load Flow Bar7/RConn3
  VI_611/RConn1 -- Pi Section Line9/LConn1 -- fault_611/LConn1
  VI_611/RConn2 -- Pi Section Line9/LConn2 -- fault_611/LConn2
  VI_611/RConn3 -- Pi Section Line9/LConn3 -- fault_611/LConn3
  Load Flow Bar9/LConn1 -- Pi Section Line12/LConn1 -- Pi Section Line9/RConn1
  Load Flow Bar9/LConn3 -- Pi Section Line12/LConn3 -- Pi Section Line9/RConn3
  Load Flow Bar9/RConn2 -- VI_684/LConn2
  Load Flow Bar9/RConn3 -- VI_684/LConn3
  Pi Section Line12/RConn1 -- VI_652/RConn1
  VI_652/RConn2 -- Pi Section Line12/RConn2
  VI_652/RConn3 -- Pi Section Line12/RConn3
  VI_652/LConn1 -- fault_652/LConn1 -- Load Flow Bar11/LConn1
  VI_652/LConn2 -- fault_652/LConn2 -- Load Flow Bar11/LConn2
  VI_652/LConn3 -- fault_652/LConn3 -- Load Flow Bar11/LConn3
  Ground10/LConn1 -- 652  Z 1/RConn1
  652  Z 2/RConn1 -- Ground11/LConn1
  Load Flow Bar11/RConn1 -- 652  Z 1/LConn1
  Load Flow Bar11/RConn2 -- "652  Z "/LConn1
  Load Flow Bar11/RConn3 -- 652  Z 2/LConn1
  VI_611/LConn1 -- Load Flow Bar10/RConn1
  VI_611/LConn2 -- Load Flow Bar10/RConn2
  VI_611/LConn3 -- Load Flow Bar10/RConn3
  611 Z1/LConn1 -- Load Flow Bar10/LConn2 -- 611 I1/LConn1
  Ground13/LConn1 -- 611 I1/RConn1
  Ground12/LConn1 -- 611 Z1/RConn1
  611 I2/LConn1 -- Load Flow Bar10/LConn1 -- 611 Z2/LConn1
  Ground14/LConn1 -- 611 Z2/RConn1
  Ground15/LConn1 -- 611 I2/RConn1
  VI_684/RConn1 -- fault_684/LConn1 -- Pi Section Line/LConn1
  VI_684/RConn2 -- fault_684/LConn2 -- Pi Section Line/LConn2
  VI_684/RConn3 -- fault_684/LConn3 -- Pi Section Line/LConn3
  646_Z1/LConn1 -- Load Flow Bar4/LConn1
  Pi Section Line5/RConn1 -- Load Flow Bar3/LConn1
  VI_646/RConn1 -- Pi Section Line5/LConn1
  671 D PQ1/LConn1 -- Load Flow Bar8/RConn1
  671 D PQ1/LConn2 -- Load Flow Bar8/RConn2
  671 D PQ1/LConn3 -- Load Flow Bar8/RConn3

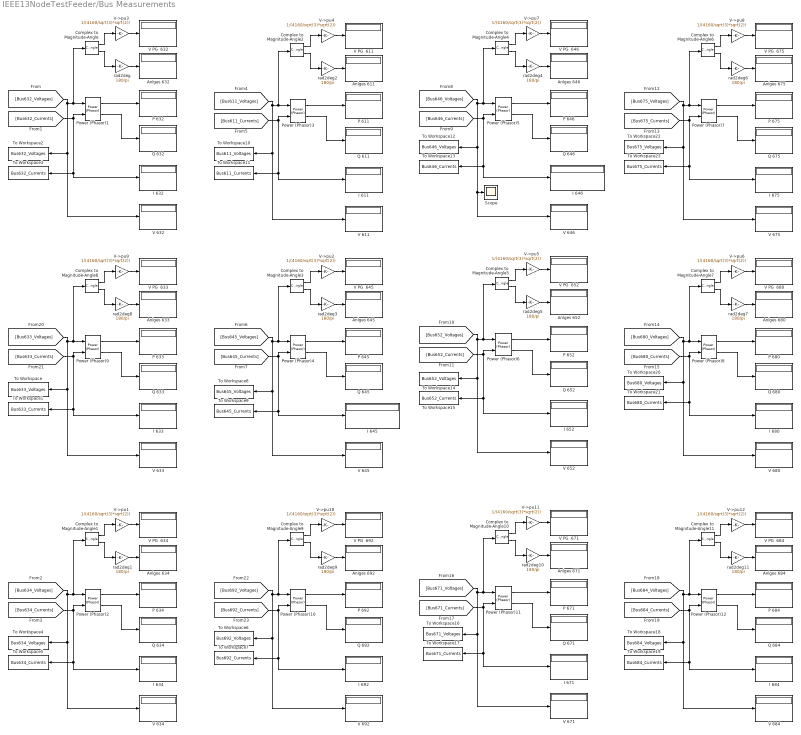
== system IEEE13NodeTestFeeder/Bus Measurements ==
  Anlges {611,632..634,645..646,652,671,675,680,684,692} (12 alike) : Display
  Complex to Magnitude-Angle{,1..11} (12 alike) : ComplexToMagnitudeAngle
  I {611,632..634,645..646,652,671,675,680,684,692} (12 alike) : Display
  P {611,632..634,645..646,652,671,675,680,684,692} (12 alike) : Display
  Power (Phasor){1..12} (12 alike) : spsPowerPhasorLib/Power (Phasor)
      settings: LibrarySourceBlock=|
      | sps_lib/Sensors and Measurements/Power
      | (Phasor)
  Q {611,632..634,645..646,652,671,675,680,684,692} (12 alike) : Display
  Scope : Scope
  To Workspace : ToWorkspace  VariableName=Bus633_Voltages  SampleTime=-1
  To Workspace1 : ToWorkspace  VariableName=Bus633_Currents  SampleTime=-1
  To Workspace10 : ToWorkspace  VariableName=Bus611_Voltages  SaveFormat=Timeseries  SampleTime=-1
  To Workspace11 : ToWorkspace  VariableName=Bus611_Currents  SaveFormat=Timeseries  SampleTime=-1
  To Workspace12 : ToWorkspace  VariableName=Bus646_Voltages  SaveFormat=Timeseries  SampleTime=-1
  To Workspace13 : ToWorkspace  VariableName=Bus646_Currents  SaveFormat=Timeseries  SampleTime=-1
  To Workspace14 : ToWorkspace  VariableName=Bus652_Voltages  SaveFormat=Timeseries  SampleTime=-1
  To Workspace15 : ToWorkspace  VariableName=Bus652_Currents  SaveFormat=Timeseries  SampleTime=-1
  To Workspace16 : ToWorkspace  VariableName=Bus671_Voltages  SaveFormat=Timeseries  SampleTime=-1
  To Workspace17 : ToWorkspace  VariableName=Bus671_Currents  SaveFormat=Timeseries  SampleTime=-1
  To Workspace18 : ToWorkspace  VariableName=Bus684_Voltages  SaveFormat=Timeseries  SampleTime=-1
  To Workspace19 : ToWorkspace  VariableName=Bus684_Currents  SaveFormat=Timeseries  SampleTime=-1
  To Workspace2 : ToWorkspace  VariableName=Bus632_Voltages  SampleTime=-1
  To Workspace20 : ToWorkspace  VariableName=Bus680_Voltages  SaveFormat=Timeseries  SampleTime=-1
  To Workspace21 : ToWorkspace  VariableName=Bus680_Currents  SaveFormat=Timeseries  SampleTime=-1
  To Workspace22 : ToWorkspace  VariableName=Bus675_Voltages  SaveFormat=Timeseries  SampleTime=-1
  To Workspace23 : ToWorkspace  VariableName=Bus675_Currents  SaveFormat=Timeseries  SampleTime=-1
  To Workspace3 : ToWorkspace  VariableName=Bus632_Currents  SampleTime=-1
  To Workspace4 : ToWorkspace  VariableName=Bus634_Voltages  SampleTime=-1
  To Workspace5 : ToWorkspace  VariableName=Bus634_Currents  SampleTime=-1
  To Workspace6 : ToWorkspace  VariableName=Bus692_Voltages  SampleTime=-1
  To Workspace7 : ToWorkspace  VariableName=Bus692_Currents  SampleTime=-1
  To Workspace8 : ToWorkspace  VariableName=Bus645_Voltages  SaveFormat=Timeseries  SampleTime=-1
  To Workspace9 : ToWorkspace  VariableName=Bus645_Currents  SaveFormat=Timeseries  SampleTime=-1
  V {611,632..634,645..646,652,671,675,680,684,692} (12 alike) : Display
  V PG  {611,632..634,645..646,652,671,675,680,684,692} (12 alike) : Display
  V->pu{1..12} (12 alike) : Gain  Gain=1/(4160/sqrt(3)*sqrt(2))
  rad2deg{,1..11} (12 alike) : Gain  Gain=180/pi
  wires:
  Power (Phasor)1/1 -> P 632/1
  Complex to Magnitude-Angle/1 -> V->pu3/1
  V->pu3/1 -> V PG  632/1
  rad2deg/1 -> Anlges 632/1
  Power (Phasor)1/2 -> Q 632/1
  Complex to Magnitude-Angle/2 -> rad2deg/1
  Complex to Magnitude-Angle1/2 -> rad2deg1/1
  Power (Phasor)2/2 -> Q 634/1
  rad2deg1/1 -> Anlges 634/1
  V->pu1/1 -> V PG  634/1
  Complex to Magnitude-Angle1/1 -> V->pu1/1
  [Bus634_Voltages] -> Power (Phasor)2/1, Complex to Magnitude-Angle1/1, To Workspace4/1, V 634/1
  Power (Phasor)2/1 -> P 634/1
  [Bus634_Currents] -> To Workspace5/1, I 634/1, Power (Phasor)2/2
  [Bus645_Currents] -> Power (Phasor)4/2, To Workspace9/1, I 645/1
  Power (Phasor)4/1 -> P 645/1
  [Bus645_Voltages] -> To Workspace8/1, V 645/1, Complex to Magnitude-Angle3/1, Power (Phasor)4/1
  Complex to Magnitude-Angle3/1 -> V->pu2/1
  V->pu2/1 -> V PG  645/1
  rad2deg3/1 -> Anlges 645/1
  Power (Phasor)4/2 -> Q 645/1
  Complex to Magnitude-Angle3/2 -> rad2deg3/1
  Complex to Magnitude-Angle2/2 -> rad2deg2/1
  Power (Phasor)3/2 -> Q 611/1
  rad2deg2/1 -> Anlges 611/1
  V->pu4/1 -> V PG  611/1
  Complex to Magnitude-Angle2/1 -> V->pu4/1
  [Bus611_Voltages] -> Power (Phasor)3/1, Complex to Magnitude-Angle2/1, To Workspace10/1, V 611/1
  Power (Phasor)3/1 -> P 611/1
  [Bus611_Currents] -> To Workspace11/1, I 611/1, Power (Phasor)3/2
  [Bus675_Currents] -> Power (Phasor)7/2, To Workspace23/1, I 675/1
  Power (Phasor)7/1 -> P 675/1
  [Bus675_Voltages] -> To Workspace22/1, V 675/1, Complex to Magnitude-Angle6/1, Power (Phasor)7/1
  Complex to Magnitude-Angle6/1 -> V->pu8/1
  V->pu8/1 -> V PG  675/1
  rad2deg6/1 -> Anlges 675/1
  Power (Phasor)7/2 -> Q 675/1
  Complex to Magnitude-Angle6/2 -> rad2deg6/1
  Complex to Magnitude-Angle7/2 -> rad2deg7/1
  Power (Phasor)8/2 -> Q 680/1
  rad2deg7/1 -> Anlges 680/1
  V->pu6/1 -> V PG  680/1
  Complex to Magnitude-Angle7/1 -> V->pu6/1
  [Bus680_Voltages] -> Power (Phasor)8/1, Complex to Magnitude-Angle7/1, To Workspace20/1, V 680/1
  Power (Phasor)8/1 -> P 680/1
  [Bus680_Currents] -> To Workspace21/1, I 680/1, Power (Phasor)8/2
  [Bus652_Currents] -> Power (Phasor)6/2, To Workspace15/1, I 652/1
  Power (Phasor)6/1 -> P 652/1
  [Bus652_Voltages] -> To Workspace14/1, V 652/1, Complex to Magnitude-Angle5/1, Power (Phasor)6/1
  Complex to Magnitude-Angle5/1 -> V->pu5/1
  V->pu5/1 -> V PG  652/1
  rad2deg5/1 -> Anlges 652/1
  Power (Phasor)6/2 -> Q 652/1
  Complex to Magnitude-Angle5/2 -> rad2deg5/1
  Complex to Magnitude-Angle4/2 -> rad2deg4/1
  Power (Phasor)5/2 -> Q 646/1
  rad2deg4/1 -> Anlges 646/1
  V->pu7/1 -> V PG  646/1
  Complex to Magnitude-Angle4/1 -> V->pu7/1
  [Bus646_Voltages] -> Power (Phasor)5/1, Complex to Magnitude-Angle4/1, To Workspace12/1, Scope/1, V 646/1
  Power (Phasor)5/1 -> P 646/1
  [Bus646_Currents] -> To Workspace13/1, I 646/1, Power (Phasor)5/2
  Complex to Magnitude-Angle10/2 -> rad2deg10/1
  Power (Phasor)11/2 -> Q 671/1
  rad2deg10/1 -> Anlges 671/1
  V->pu11/1 -> V PG  671/1
  Complex to Magnitude-Angle10/1 -> V->pu11/1
  [Bus671_Voltages] -> Power (Phasor)11/1, Complex to Magnitude-Angle10/1, To Workspace16/1, V 671/1
  Power (Phasor)11/1 -> P 671/1
  [Bus671_Currents] -> To Workspace17/1, I 671/1, Power (Phasor)11/2
  [Bus684_Currents] -> Power (Phasor)12/2, To Workspace19/1, I 684/1
  Power (Phasor)12/1 -> P 684/1
  [Bus684_Voltages] -> To Workspace18/1, V 684/1, Complex to Magnitude-Angle11/1, Power (Phasor)12/1
  Complex to Magnitude-Angle11/1 -> V->pu12/1
  V->pu12/1 -> V PG  684/1
  rad2deg11/1 -> Anlges 684/1
  Power (Phasor)12/2 -> Q 684/1
  Complex to Magnitude-Angle11/2 -> rad2deg11/1
  Complex to Magnitude-Angle9/2 -> rad2deg9/1
  Power (Phasor)10/2 -> Q 692/1
  rad2deg9/1 -> Anlges 692/1
  V->pu10/1 -> V PG  692/1
  Complex to Magnitude-Angle9/1 -> V->pu10/1
  [Bus692_Voltages] -> Power (Phasor)10/1, Complex to Magnitude-Angle9/1, To Workspace6/1, V 692/1
  Power (Phasor)10/1 -> P 692/1
  [Bus692_Currents] -> To Workspace7/1, I 692/1, Power (Phasor)10/2
  [Bus633_Currents] -> Power (Phasor)9/2, I 633/1, To Workspace1/1
  Power (Phasor)9/1 -> P 633/1
  [Bus633_Voltages] -> To Workspace/1, V 633/1, Complex to Magnitude-Angle8/1, Power (Phasor)9/1
  Complex to Magnitude-Angle8/1 -> V->pu9/1
  V->pu9/1 -> V PG  633/1
  rad2deg8/1 -> Anlges 633/1
  Power (Phasor)9/2 -> Q 633/1
  Complex to Magnitude-Angle8/2 -> rad2deg8/1
  [Bus632_Voltages] -> To Workspace2/1, V 632/1, Complex to Magnitude-Angle/1, Power (Phasor)1/1
  [Bus632_Currents] -> Power (Phasor)1/2, To Workspace3/1, I 632/1

== system IEEE13NodeTestFeeder/Double click here for more info ==

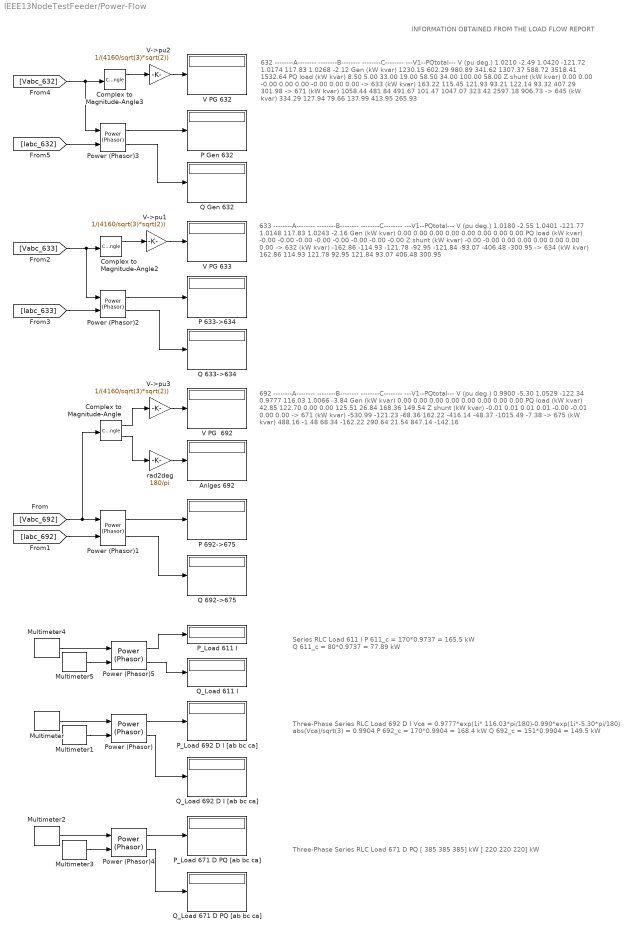
== system IEEE13NodeTestFeeder/Power-Flow ==
  note: 692 --------A-------- --------B-------- --------C-------- ---V1--PQtotal---
      | V (pu deg.) 0.9900 -5.30 1.0529 -122.34 0.9777 116.03 1.0066 -3.84
      | Gen (kW kvar) 0.00 0.00 0.00 0.00 0.00 0.00 0.00 0.00
      | PQ load (kW kvar) 42.85 122.70 0.00 0.00 125.51 26.84 168.36 149.54
      | Z shunt (kW kvar) -0.01 0.01 0.01 0.01 -0.00 -0.01 0.00 0.00
      |
      | -> 671 (kW kvar) -530.99 -121.23 -68.36 162.22 -416.14 -48.37 -1015.49 -7.38
      | -> 675 (kW kvar) 488.16 -1.48 68.34 -162.22 290.64 21.54 847.14 -142.16
  note: 633 --------A-------- --------B-------- --------C-------- ---V1--PQtotal---
      | V (pu deg.) 1.0180 -2.55 1.0401 -121.77 1.0148 117.83 1.0243 -2.16
      | Gen (kW kvar) 0.00 0.00 0.00 0.00 0.00 0.00 0.00 0.00
      | PQ load (kW kvar) -0.00 -0.00 -0.00 -0.00 -0.00 -0.00 -0.00 -0.00
      | Z shunt (kW kvar) -0.00 -0.00 0.00 0.00 0.00 0.00 0.00 0.00
      |
      | -> 632 (kW kvar) -162.86 -114.93 -121.78 -92.95 -121.84 -93.07 -406.48 -300.95
      | -> 634 (kW kvar) 162.86 114.93 121.78 92.95 121.84 93.07 406.48 300.95
  note: 632 --------A-------- --------B-------- --------C-------- ---V1--PQtotal---
      | V (pu deg.) 1.0210 -2.49 1.0420 -121.72 1.0174 117.83 1.0268 -2.12
      | Gen (kW kvar) 1230.15 602.29 980.89 341.62 1307.37 588.72 3518.41 1532.64
      | PQ load (kW kvar) 8.50 5.00 33.00 19.00 58.50 34.00 100.00 58.00
      | Z shunt (kW kvar) 0.00 0.00 -0.00 0.00 0.00 -0.00 0.00 0.00
      |
      | -> 633 (kW kvar) 163.22 115.45 121.93 93.21 122.14 93.32 407.29 301.98
      | -> 671 (kW kvar) 1058.44 481.84 491.67 101.47 1047.07 323.42 2597.18 906.73
      | -> 645 (kW kvar) 334.29 127.94 79.66 137.99 413.95 265.93
  note: Three-Phase Series RLC Load 671 D PQ
      | [ 385 385 385] kW
      | [ 220 220 220] kW
  note: Three-Phase Series RLC Load 692 D I
      | Vca = 0.9777*exp(1i* 116.03*pi/180)-0.990*exp(1i*-5.30*pi/180)
      | abs(Vca)/sqrt(3) = 0.9904
      | P 692_c = 170*0.9904 = 168.4 kW
      | Q 692_c = 151*0.9904 = 149.5 kW
  note: Series RLC Load 611 I
      | P 611_c = 170*0.9737 = 165.5 kW
      | Q 611_c = 80*0.9737 = 77.89 kW
  note: INFORMATION OBTAINED FROM THE LOAD FLOW REPORT
  Anlges 692 : Display
  Complex to Magnitude-Angle : ComplexToMagnitudeAngle
  Complex to Magnitude-Angle2 : ComplexToMagnitudeAngle
  Complex to Magnitude-Angle3 : ComplexToMagnitudeAngle
  Multimeter : spsMultimeterLib/Multimeter  L=30  sel=[11 12 13]  yselected={}  Gain=[1 1 1]  OutputType=Complex  PlotAtSimulationStop=off  PhasorSimulation=on
  Multimeter1 : spsMultimeterLib/Multimeter  L=30  sel=[21 25 26]  yselected={}  Gain=[1 1 1]  OutputType=Complex  PlotAtSimulationStop=off  PhasorSimulation=on
  Multimeter2 : spsMultimeterLib/Multimeter  L=30  sel=[2 3 4]  yselected={}  Gain=[1 1 1]  OutputType=Complex  PlotAtSimulationStop=off  PhasorSimulation=on
  Multimeter3 : spsMultimeterLib/Multimeter  L=30  sel=[15 16 17]  yselected={}  Gain=[1 1 1]  OutputType=Complex  PlotAtSimulationStop=off  PhasorSimulation=on
  Multimeter4 : spsMultimeterLib/Multimeter  L=30  sel=1  yselected={}  Gain=1  OutputType=Complex  PlotAtSimulationStop=off  PhasorSimulation=on
  Multimeter5 : spsMultimeterLib/Multimeter  L=30  sel=14  yselected={}  Gain=1  OutputType=Complex  PlotAtSimulationStop=off  PhasorSimulation=on
  P 633->634 : Display
  P 692->675 : Display
  P Gen 632 : Display
  P_Load 611 I : Display
  P_Load 671 D PQ [ab bc ca] : Display
  P_Load 692 D I [ab bc ca] : Display
  Power (Phasor){,1..5} (6 alike) : spsPowerPhasorLib/Power (Phasor)
      settings: LibrarySourceBlock=|
      | sps_lib/Sensors and Measurements/Power
      | (Phasor)
  Q 633->634 : Display
  Q 692->675 : Display
  Q Gen 632 : Display
  Q_Load 611 I : Display
  Q_Load 671 D PQ [ab bc ca] : Display
  Q_Load 692 D I [ab bc ca] : Display
  V PG  692 : Display
  V PG 632 : Display
  V PG 633 : Display
  V->pu1 : Gain  Gain=1/(4160/sqrt(3)*sqrt(2))
  V->pu2 : Gain  Gain=1/(4160/sqrt(3)*sqrt(2))
  V->pu3 : Gain  Gain=1/(4160/sqrt(3)*sqrt(2))
  rad2deg : Gain  Gain=180/pi
  wires:
  V->pu3/1 -> V PG  692/1
  Power (Phasor)5/2 -> Q_Load 611 I/1
  Power (Phasor)5/1 -> P_Load 611 I/1
  Multimeter5/1 -> Power (Phasor)5/2
  Multimeter4/1 -> Power (Phasor)5/1
  rad2deg/1 -> Anlges 692/1
  Complex to Magnitude-Angle/2 -> rad2deg/1
  [Vabc_692] -> Complex to Magnitude-Angle/1, Power (Phasor)1/1
  Complex to Magnitude-Angle/1 -> V->pu3/1
  Power (Phasor)4/2 -> Q_Load 671 D PQ [ab bc ca]/1
  Power (Phasor)4/1 -> P_Load 671 D PQ [ab bc ca]/1
  Multimeter3/1 -> Power (Phasor)4/2
  Multimeter2/1 -> Power (Phasor)4/1
  Power (Phasor)/2 -> Q_Load 692 D I [ab bc ca]/1
  Power (Phasor)/1 -> P_Load 692 D I [ab bc ca]/1
  Multimeter1/1 -> Power (Phasor)/2
  Multimeter/1 -> Power (Phasor)/1
  V->pu2/1 -> V PG 632/1
  [Vabc_632] -> Complex to Magnitude-Angle3/1, Power (Phasor)3/1
  Complex to Magnitude-Angle3/1 -> V->pu2/1
  Power (Phasor)3/2 -> Q Gen 632/1
  Power (Phasor)3/1 -> P Gen 632/1
  [Iabc_632] -> Power (Phasor)3/2
  V->pu1/1 -> V PG 633/1
  [Vabc_633] -> Complex to Magnitude-Angle2/1, Power (Phasor)2/1
  Complex to Magnitude-Angle2/1 -> V->pu1/1
  Power (Phasor)2/2 -> Q 633->634/1
  Power (Phasor)2/1 -> P 633->634/1
  [Iabc_633] -> Power (Phasor)2/2
  Power (Phasor)1/2 -> Q 692->675/1
  Power (Phasor)1/1 -> P 692->675/1
  [Iabc_692] -> Power (Phasor)1/2
